simulink model "fxpdemo_lookup_shared_param"  (Simulink 7.6)
settings: Solver=FixedStepDiscrete  StartTime=0.0  StopTime=10.0  FixedStep=1  RelTol=1e-3
PreLoadFcn:
  | tabledata=Simulink.Parameter;
  | tabledata.RTWInfo.StorageClass = 'ExportedGlobal';
  | tabledata.DataType='fixdt(0,8,6)';
  | tabledata.Value=sin(linspace(0,pi,10));
Description:
  | Sharing Parameters in Prelookup and Interpolation Blocks
  | The Prelookup and Interpolation Using Prelookup blocks have support for specifying
  | the data type for the breakpoints and table parameters. This makes it possible
  | for blocks that have different port data types to share their parameter data in the
  | generated code. One way of doing this is to specify the parameter with the same
  | values and data types in multiple blocks. This is done in the Prelookup blocks in this
  | model. Another way is to use a Simulink.Parameter object to define the blocks'
  | shared parameter. This is done for the Interpolation blocks. The *Table data type*
  | must be set to: |Inherit: Inherit from 'Table data'|.
  | 
  | For parameter sharing to take effect, the *Inline parameters* check box must be
  | selected in the Optimization pane of the Configuration Parameters dialog box.
  | 
  | To see this in the generated code, open the model and build it.
CloseFcn:
  | clear tabledata;
settings Model: Creator=The MathWorks Inc.
settings DataIOCC: SaveFormat=StructureWithTime
settings OptimizationCC: InlineParams=on
settings DebuggingCC: ParameterPrecisionLossMsg=none  StrictBusMsg=Warning
settings RTWCC: GenCodeOnly=on  GenerateReport=on  RTWVerbose=off  ProcessScript=grt_make_rtw_hook  LaunchReport=on

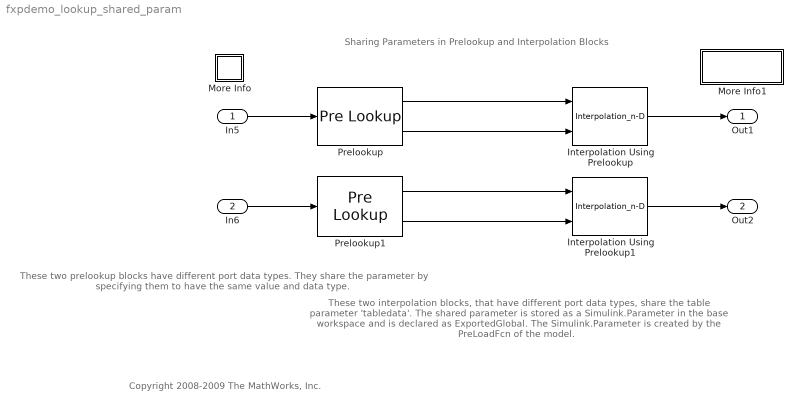
== system fxpdemo_lookup_shared_param ==
  note: Copyright 2008-2009 The MathWorks, Inc.
  note: These two interpolation blocks, that have different
      | port data types, share the table parameter 'tabledata'.
      | The shared parameter is stored as a Simulink.Parameter
      | in the base workspace and is declared as ExportedGlobal.
      |
      | The Simulink.Parameter is created by the PreLoadFcn of
      | the model.
  note: These two prelookup blocks have different port
      | data types. They share the parameter by specifying
      | them to have the same value and data type.
  note: Sharing Parameters in Prelookup and Interpolation Blocks
  In5 : Inport  OutDataTypeStr=fixdt(1,16,2^-5,0)
  In6 : Inport  Port=2  OutDataTypeStr=fixdt(1,16,2^-8,0)
  Interpolation Using Prelookup : Interpolation_n-D  NumberOfTableDimensions=1  Table=tabledata  ExtrapMethod=None - Clip  CheckIndexInCode=off  OutDataTypeStr=fixdt(1,16,2^-8,0)  TableDataTypeStr=Inherit: Inherit from 'Table data'
      settings: InputPortMap=u0,u1
  Interpolation Using Prelookup1 : Interpolation_n-D  NumberOfTableDimensions=1  Table=tabledata  ExtrapMethod=None - Clip  CheckIndexInCode=off  OutDataTypeStr=fixdt(1,16,2^-4,0)  TableDataTypeStr=Inherit: Inherit from 'Table data'
      settings: InputPortMap=u0,u1
  More Info : Subsystem
      settings: OpenFcn=showdemo(bdroot(gcs))
      mask Display: disp('?')
  More Info1 : Subsystem
      settings: OpenFcn=rtwbuild(bdroot(gcs))
      mask Display: fprintf('Double-click to\ngenerate code')
  Prelookup : PreLookup  BreakpointsData=exp(linspace(1,3,10))  BreakpointDataTypeStr=fixdt(1,16,10)  FractionDataTypeStr=fixdt(1,16,14)
  Prelookup1 : PreLookup  BreakpointsData=exp(linspace(1,3,10))  BreakpointDataTypeStr=fixdt(1,16,10)  FractionDataTypeStr=fixdt(0,8,7)
      settings: LockScale=on
  Out1 : Outport
  Out2 : Outport  Port=2
  wires:
  Interpolation Using Prelookup/1 -> Out1/1
  Interpolation Using Prelookup1/1 -> Out2/1
  In5/1 -> Prelookup/1
  In6/1 -> Prelookup1/1
  Prelookup/1 -> Interpolation Using Prelookup/1
  Prelookup/2 -> Interpolation Using Prelookup/2
  Prelookup1/1 -> Interpolation Using Prelookup1/1
  Prelookup1/2 -> Interpolation Using Prelookup1/2

== system fxpdemo_lookup_shared_param/More Info ==

== system fxpdemo_lookup_shared_param/More Info1 ==
